simulink model "AM5_1"  (R2020b)
settings: Solver=VariableStepDiscrete  StartTime=0.0  StopTime=2  MaxStep=1/800  RelTol=1e-3
settings Model: Creator=seojoon  LastModifiedBy=seojoon

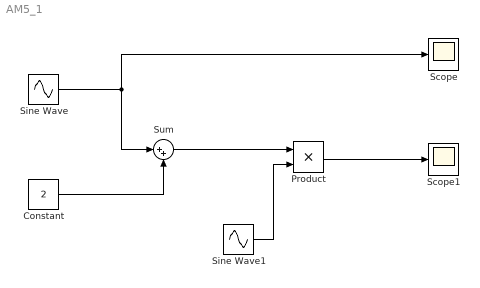
== system AM5_1 ==
  Constant : Constant  Value=2
  Product : Product
  Scope : Scope
  Scope1 : Scope
  Sine Wave : Sin  Amplitude=2  Frequency=2*pi*5  SampleTime=0
  Sine Wave1 : Sin  Frequency=2*pi*50  Phase=pi/2  SampleTime=0
  Sum : Sum  Inputs=|++
  wires:
  Sine Wave/1 -> Sum/1, Scope/1
  Constant/1 -> Sum/2
  Sum/1 -> Product/1
  Sine Wave1/1 -> Product/2
  Product/1 -> Scope1/1
